simulink model "IEEE14_case"  (R2024b)
settings: Solver=FixedStepAuto  StartTime=0  StopTime=2  FixedStep=1e-7  RelTol=1e-3
values from neighbouring files (symbols this model uses):
  GFL_15_Bva = 0.009    [IEEE14_parameters.m]
  GFL_15_C_bus_pu = 7.179419    [IEEE14_parameters.m]
  GFL_15_f0 = 60    [IEEE14_parameters.m]
  GFL_15_I_id = 691.26967    [IEEE14_parameters.m]
  GFL_15_I_iq = 691.26967    [IEEE14_parameters.m]
  GFL_15_I_od = 45.2207    [IEEE14_parameters.m]
  GFL_15_I_oq = 45.2207    [IEEE14_parameters.m]
  GFL_15_I_pll = 0.78    [IEEE14_parameters.m]
  GFL_15_Kdi = 0.09    [IEEE14_parameters.m]
  GFL_15_Kdo = 0.9    [IEEE14_parameters.m]
  GFL_15_Kqi = 0.09    [IEEE14_parameters.m]
  GFL_15_Kqo = 0.9    [IEEE14_parameters.m]
  GFL_15_Lg_pu = 0.631447    [IEEE14_parameters.m]
  GFL_15_mode = 1    [IEEE14_parameters.m]
  GFL_15_P_id = 3.7166    [IEEE14_parameters.m]
  GFL_15_P_iq = 3.7166    [IEEE14_parameters.m]
  GFL_15_P_od = 0.4798    [IEEE14_parameters.m]
  GFL_15_P_oq = 0.4798    [IEEE14_parameters.m]
  GFL_15_P_pll = 290.42    [IEEE14_parameters.m]
  GFL_15_Qe_ref = 0.2    [IEEE14_parameters.m]
  GFL_15_Rg_pu = 0.024016    [IEEE14_parameters.m]
  GFL_15_Sbase = 1.000000e+4    (= 10000)    [IEEE14_parameters.m]
  GFL_15_Tdi = 0.01    [IEEE14_parameters.m]
  GFL_15_Tdo = 0.2    [IEEE14_parameters.m]
  GFL_15_Tqi = 0.01    [IEEE14_parameters.m]
  GFL_15_Tqo = 0.2    [IEEE14_parameters.m]
  GFL_15_Vbase = 380    [IEEE14_parameters.m]
  GFL_15_Vdc_ref = 1.011475    [IEEE14_parameters.m]
  GFL_15_Vdcbase = 700    [IEEE14_parameters.m]
  GFL_15_vq_ref = 0    [IEEE14_parameters.m]
  GFL_16_Bva = 0.002    [IEEE14_parameters.m]
  GFL_16_C_bus_pu = 7.179419    [IEEE14_parameters.m]
  GFL_16_f0 = 60    [IEEE14_parameters.m]
  GFL_16_I_id = 691.26967    [IEEE14_parameters.m]
  GFL_16_I_iq = 691.26967    [IEEE14_parameters.m]
  GFL_16_I_od = 45.2207    [IEEE14_parameters.m]
  GFL_16_I_oq = 45.2207    [IEEE14_parameters.m]
  GFL_16_I_pll = 0.78    [IEEE14_parameters.m]
  GFL_16_Kdi = 0.05    [IEEE14_parameters.m]
  GFL_16_Kdo = 0.5    [IEEE14_parameters.m]
  GFL_16_Kqi = 0.05    [IEEE14_parameters.m]
  GFL_16_Kqo = 0.5    [IEEE14_parameters.m]
  GFL_16_Lg_pu = 0.631447    [IEEE14_parameters.m]
  GFL_16_mode = 1    [IEEE14_parameters.m]
  GFL_16_P_id = 3.7166    [IEEE14_parameters.m]
  GFL_16_P_iq = 3.7166    [IEEE14_parameters.m]
  GFL_16_P_od = 0.4798    [IEEE14_parameters.m]
  GFL_16_P_oq = 0.4798    [IEEE14_parameters.m]
  GFL_16_P_pll = 290.42    [IEEE14_parameters.m]
  GFL_16_Qe_ref = 0.2    [IEEE14_parameters.m]
  GFL_16_Rg_pu = 0.024016    [IEEE14_parameters.m]
  GFL_16_Sbase = 1.000000e+4    (= 10000)    [IEEE14_parameters.m]
  GFL_16_Tdi = 0.01    [IEEE14_parameters.m]
  GFL_16_Tdo = 0.2    [IEEE14_parameters.m]
  GFL_16_Tqi = 0.01    [IEEE14_parameters.m]
  GFL_16_Tqo = 0.2    [IEEE14_parameters.m]
  GFL_16_Vbase = 380    [IEEE14_parameters.m]
  GFL_16_Vdc_ref = 1.01144    [IEEE14_parameters.m]
  GFL_16_Vdcbase = 700    [IEEE14_parameters.m]
  GFL_16_vq_ref = 0    [IEEE14_parameters.m]
  GFL_17_Bva = 0.002    [IEEE14_parameters.m]
  GFL_17_C_bus_pu = 7.179419    [IEEE14_parameters.m]
  GFL_17_f0 = 60    [IEEE14_parameters.m]
  GFL_17_I_id = 691.26967    [IEEE14_parameters.m]
  GFL_17_I_iq = 691.26967    [IEEE14_parameters.m]
  GFL_17_I_od = 45.2207    [IEEE14_parameters.m]
  GFL_17_I_oq = 45.2207    [IEEE14_parameters.m]
  GFL_17_I_pll = 0.78    [IEEE14_parameters.m]
  GFL_17_Kdi = 0.05    [IEEE14_parameters.m]
  GFL_17_Kdo = 0.5    [IEEE14_parameters.m]
  GFL_17_Kqi = 0.05    [IEEE14_parameters.m]
  GFL_17_Kqo = 0.5    [IEEE14_parameters.m]
  GFL_17_Lg_pu = 0.631447    [IEEE14_parameters.m]
  GFL_17_mode = 1    [IEEE14_parameters.m]
  GFL_17_P_id = 3.7166    [IEEE14_parameters.m]
  GFL_17_P_iq = 3.7166    [IEEE14_parameters.m]
  GFL_17_P_od = 0.4798    [IEEE14_parameters.m]
  GFL_17_P_oq = 0.4798    [IEEE14_parameters.m]
  GFL_17_P_pll = 290.42    [IEEE14_parameters.m]
  GFL_17_Qe_ref = 0.2    [IEEE14_parameters.m]
  GFL_17_Rg_pu = 0.024016    [IEEE14_parameters.m]
  GFL_17_Sbase = 1.000000e+4    (= 10000)    [IEEE14_parameters.m]
  GFL_17_Tdi = 0.01    [IEEE14_parameters.m]
  GFL_17_Tdo = 0.2    [IEEE14_parameters.m]
  GFL_17_Tqi = 0.01    [IEEE14_parameters.m]
  GFL_17_Tqo = 0.2    [IEEE14_parameters.m]
  GFL_17_Vbase = 380    [IEEE14_parameters.m]
  GFL_17_Vdc_ref = 1.011632    [IEEE14_parameters.m]
  GFL_17_Vdcbase = 700    [IEEE14_parameters.m]
  GFL_17_vq_ref = 0    [IEEE14_parameters.m]
  GFL_18_Bva = 0.002    [IEEE14_parameters.m]
  GFL_18_C_bus_pu = 7.179419    [IEEE14_parameters.m]
  GFL_18_f0 = 60    [IEEE14_parameters.m]
  GFL_18_I_id = 691.26967    [IEEE14_parameters.m]
  GFL_18_I_iq = 691.26967    [IEEE14_parameters.m]
  GFL_18_I_od = 45.2207    [IEEE14_parameters.m]
  GFL_18_I_oq = 45.2207    [IEEE14_parameters.m]
  GFL_18_I_pll = 0.78    [IEEE14_parameters.m]
  GFL_18_Kdi = 0.05    [IEEE14_parameters.m]
  GFL_18_Kdo = 0.5    [IEEE14_parameters.m]
  GFL_18_Kqi = 0.05    [IEEE14_parameters.m]
  GFL_18_Kqo = 0.5    [IEEE14_parameters.m]
  GFL_18_Lg_pu = 0.631447    [IEEE14_parameters.m]
  GFL_18_mode = 1    [IEEE14_parameters.m]
  GFL_18_P_id = 3.7166    [IEEE14_parameters.m]
  GFL_18_P_iq = 3.7166    [IEEE14_parameters.m]
  GFL_18_P_od = 0.4798    [IEEE14_parameters.m]
  GFL_18_P_oq = 0.4798    [IEEE14_parameters.m]
  GFL_18_P_pll = 290.42    [IEEE14_parameters.m]
  GFL_18_Qe_ref = 0.2    [IEEE14_parameters.m]
  GFL_18_Rg_pu = 0.024016    [IEEE14_parameters.m]
  GFL_18_Sbase = 1.000000e+4    (= 10000)    [IEEE14_parameters.m]
  GFL_18_Tdi = 0.01    [IEEE14_parameters.m]
  GFL_18_Tdo = 0.2    [IEEE14_parameters.m]
  GFL_18_Tqi = 0.01    [IEEE14_parameters.m]
  GFL_18_Tqo = 0.2    [IEEE14_parameters.m]
  GFL_18_Vbase = 380    [IEEE14_parameters.m]
  GFL_18_Vdc_ref = 1.011572    [IEEE14_parameters.m]
  GFL_18_Vdcbase = 700    [IEEE14_parameters.m]
  GFL_18_vq_ref = 0    [IEEE14_parameters.m]
  ... (+180 more)
(part 22 of 25)

== system IEEE14_case/SG_D_6/d_psi_fd_SG_D_6_block ==
  note: d_psi_fd_SG_D_6 in case14gfl
      | $-\frac{\psi _{\mathrm{fd},\mathrm{SG},D,6}-E_{\mathrm{fd},\mathrm{SG},D,6}+\left(x_{d}-x_{\mathrm{dd}}\right)\,\left(\frac{\frac{\psi _{\mathrm{1d},\mathrm{SG},D,6}\,\left(x_{\mathrm{dd}}-x_{\mathrm{ddd}}\right)}{x_{\mathrm{dd}}-x_{l}}-\psi _{d,\mathrm{SG},D,6}+\frac{\psi _{\mathrm{fd},\mathrm{SG},D,6}\,\left(x_{\mathrm{ddd}}-x_{l}\right)}{x_{\mathrm{dd}}-x_{l}}}{x_{\mathrm{ddd}}}-\frac{\left(x_{\mathrm{dd}}-x_{\mathrm{ddd}}\right)\,\left(\psi _{\mathrm{1d},\mathrm{SG},D,6}-\psi _{\mathrm{fd},\mathrm{SG},D,6}+\frac{\left(x_{\mathrm{dd}}-x_{l}\right)\,\left(\frac{\psi _{\mathrm{1d},\mathrm{SG},D,6}\,\left(x_{\mathrm{dd}}-x_{\mathrm{ddd}}\right)}{x_{\mathrm{dd}}-x_{l}}-\psi _{d,\mathrm{SG},D,6}+\frac{\psi _{\mathrm{fd},\mathrm{SG},D,6}\,\left(x_{\mathrm{ddd}}-x_{l}\right)}{x_{\mathrm{dd}}-x_{l}}\right)}{x_{\mathrm{ddd}}}\right)}{{\left(x_{\mathrm{dd}}-x_{l}\right)}^2}\right)}{T_{\mathrm{dd}}}$
      | Automatically generated on 2025-10-09 21:32:58 .
  State_E_fd_SG_D_6_8c2c7 : Inport
  State_psi_fd_SG_D_6_cff00 : Inport  Port=2
  State_psi_1d_SG_D_6_bc672 : Inport  Port=3
  State_psi_fd_SG_D_6_4e3f4 : Inport  Port=4
  State_psi_1d_SG_D_6_ebde4 : Inport  Port=5
  State_psi_d_SG_D_6_92222 : Inport  Port=6
  State_psi_fd_SG_D_6_38b04 : Inport  Port=7
  State_psi_1d_SG_D_6_32df7 : Inport  Port=8
  State_psi_d_SG_D_6_beaed : Inport  Port=9
  State_psi_fd_SG_D_6_10d72 : Inport  Port=10
  Add_ba2f2 : Sum
  Add_cdb5d : Sum
  Constant_-1_792aa : Constant  Value=-1
  Constant_-1_a3724 : Constant  Value=-1
  Constant_-1_f4132 : Constant  Value=-1
  Constant_2.0_0b013 : Constant  Value=2.0
  Constant_T_dd_62463 : Constant  Value=T_dd
  Constant_x_d_b318c : Constant  Value=x_d
  Constant_x_dd_0a587 : Constant  Value=x_dd
  Constant_x_dd_2d805 : Constant  Value=x_dd
  Constant_x_dd_68d39 : Constant  Value=x_dd
  Constant_x_dd_81c4f : Constant  Value=x_dd
  Constant_x_dd_82b55 : Constant  Value=x_dd
  Constant_x_dd_8a32d : Constant  Value=x_dd
  Constant_x_dd_b822f : Constant  Value=x_dd
  Constant_x_dd_ddb07 : Constant  Value=x_dd
  Constant_x_dd_f11c0 : Constant  Value=x_dd
  Constant_x_dd_fd22e : Constant  Value=x_dd
  Constant_x_ddd_04df1 : Constant  Value=x_ddd
  Constant_x_ddd_0bc83 : Constant  Value=x_ddd
  Constant_x_ddd_0c2e6 : Constant  Value=x_ddd
  Constant_x_ddd_68b46 : Constant  Value=x_ddd
  Constant_x_ddd_9c9d7 : Constant  Value=x_ddd
  Constant_x_ddd_b1a79 : Constant  Value=x_ddd
  Constant_x_ddd_f3fb2 : Constant  Value=x_ddd
  Constant_x_l_2e508 : Constant  Value=x_l
  Constant_x_l_329a5 : Constant  Value=x_l
  Constant_x_l_400bf : Constant  Value=x_l
  Constant_x_l_84374 : Constant  Value=x_l
  Constant_x_l_978cf : Constant  Value=x_l
  Constant_x_l_b454b : Constant  Value=x_l
  Constant_x_l_d1dca : Constant  Value=x_l
  Constant_x_l_deb57 : Constant  Value=x_l
  Divide_172f0 : Product  Inputs=*/
  Divide_302a3 : Product  Inputs=*/
  Divide_32902 : Product  Inputs=*/
  Divide_a0797 : Product  Inputs=*/
  Divide_ab6db : Product  Inputs=*/
  Divide_b1b26 : Product  Inputs=*/
  Divide_d407a : Product  Inputs=*/
  Divide_da2d9 : Product  Inputs=*/
  Power_b35c3 : Math  Operator=pow
  Product_04d90 : Product
  Product_25107 : Product
  Product_3678f : Product
  Product_38c26 : Product
  Product_4f01a : Product
  Product_8b753 : Product
  Product_9bbf1 : Product
  Product_adb41 : Product
  Product_f7c34 : Product
  Product_fcd24 : Product
  Subtract_088af : Sum  Inputs=+-
  Subtract_0a0c0 : Sum  Inputs=+-
  Subtract_0b103 : Sum  Inputs=+-
  Subtract_121da : Sum  Inputs=+-
  Subtract_441e5 : Sum  Inputs=+-
  Subtract_539cc : Sum  Inputs=+-
  Subtract_59274 : Sum  Inputs=+-
  Subtract_66fab : Sum  Inputs=+-
  Subtract_6b641 : Sum  Inputs=+-
  Subtract_8929d : Sum  Inputs=+-
  Subtract_8cd83 : Sum  Inputs=+-
  Subtract_8e7ae : Sum  Inputs=+-
  Subtract_923ad : Sum  Inputs=+-
  Subtract_9258f : Sum  Inputs=+-
  Subtract_960a4 : Sum  Inputs=+-
  Subtract_a221f : Sum  Inputs=+-
  Subtract_bcf8f : Sum  Inputs=+-
  Subtract_daa8f : Sum  Inputs=+-
  Subtract_e7b9f : Sum  Inputs=+-
  Blockout_d_psi_fd_SG_D_6_50674 : Outport
  wires:
  Constant_-1_a3724/1 -> Product_8b753/1
  Constant_x_l_329a5/1 -> Subtract_121da/2
  Constant_x_dd_0a587/1 -> Subtract_0a0c0/1
  State_psi_1d_SG_D_6_ebde4/1 -> Product_8b753/2
  Constant_x_dd_8a32d/1 -> Subtract_088af/1
  Subtract_59274/1 -> Product_25107/2
  Constant_x_ddd_b1a79/1 -> Subtract_0a0c0/2
  Constant_-1_792aa/1 -> Product_9bbf1/1
  Product_8b753/1 -> Product_f7c34/1
  Constant_x_dd_b822f/1 -> Subtract_0b103/1
  Constant_x_l_978cf/1 -> Subtract_66fab/2
  Subtract_0a0c0/1 -> Product_f7c34/2
  Constant_x_l_2e508/1 -> Subtract_088af/2
  Subtract_960a4/1 -> Product_adb41/2
  Constant_x_ddd_0bc83/1 -> Subtract_960a4/1
  Constant_x_l_deb57/1 -> Subtract_960a4/2
  Product_f7c34/1 -> Divide_d407a/1
  Constant_x_dd_2d805/1 -> Subtract_9258f/1
  Subtract_088af/1 -> Divide_d407a/2
  State_psi_fd_SG_D_6_38b04/1 -> Product_adb41/1
  Subtract_8e7ae/1 -> Product_3678f/1
  Constant_x_dd_f11c0/1 -> Subtract_121da/1
  Constant_T_dd_62463/1 -> Divide_32902/2
  State_psi_1d_SG_D_6_bc672/1 -> Subtract_e7b9f/1
  Divide_d407a/1 -> Add_cdb5d/1
  Product_38c26/1 -> Divide_302a3/1
  Divide_172f0/1 -> Subtract_8cd83/2
  State_psi_d_SG_D_6_92222/1 -> Add_cdb5d/2
  Product_adb41/1 -> Divide_172f0/1
  Subtract_121da/1 -> Divide_172f0/2
  Constant_x_dd_68d39/1 -> Subtract_8e7ae/1
  Constant_x_l_84374/1 -> Subtract_8e7ae/2
  Add_cdb5d/1 -> Subtract_8cd83/1
  Subtract_e7b9f/1 -> Subtract_539cc/1
  State_psi_1d_SG_D_6_32df7/1 -> Product_9bbf1/2
  Constant_x_ddd_0c2e6/1 -> Subtract_0b103/2
  Subtract_8cd83/1 -> Product_3678f/2
  Product_9bbf1/1 -> Product_4f01a/1
  Subtract_0b103/1 -> Product_4f01a/2
  Subtract_441e5/1 -> Product_38c26/2
  Constant_x_l_b454b/1 -> Subtract_9258f/2
  Constant_x_ddd_68b46/1 -> Subtract_441e5/1
  Constant_x_l_400bf/1 -> Subtract_441e5/2
  State_psi_d_SG_D_6_beaed/1 -> Add_ba2f2/2
  Constant_x_dd_ddb07/1 -> Subtract_59274/1
  Constant_x_ddd_f3fb2/1 -> Subtract_59274/2
  Constant_x_dd_fd22e/1 -> Subtract_8929d/1
  State_psi_fd_SG_D_6_4e3f4/1 -> Subtract_e7b9f/2
  Product_3678f/1 -> Divide_ab6db/1
  Constant_x_ddd_9c9d7/1 -> Divide_ab6db/2
  Product_4f01a/1 -> Divide_da2d9/1
  Subtract_9258f/1 -> Divide_da2d9/2
  State_psi_fd_SG_D_6_10d72/1 -> Product_38c26/1
  Constant_x_dd_82b55/1 -> Subtract_66fab/1
  Constant_-1_f4132/1 -> Product_25107/1
  Divide_ab6db/1 -> Subtract_539cc/2
  Product_25107/1 -> Product_fcd24/1
  Divide_da2d9/1 -> Add_ba2f2/1
  Constant_x_l_d1dca/1 -> Subtract_8929d/2
  Subtract_66fab/1 -> Divide_302a3/2
  Subtract_539cc/1 -> Product_fcd24/2
  Subtract_8929d/1 -> Power_b35c3/1
  Constant_2.0_0b013/1 -> Power_b35c3/2
  Add_ba2f2/1 -> Subtract_bcf8f/1
  Divide_302a3/1 -> Subtract_bcf8f/2
  Product_fcd24/1 -> Divide_b1b26/1
  Power_b35c3/1 -> Divide_b1b26/2
  Subtract_bcf8f/1 -> Divide_a0797/1
  Constant_x_ddd_04df1/1 -> Divide_a0797/2
  Constant_x_d_b318c/1 -> Subtract_daa8f/1
  Constant_x_dd_81c4f/1 -> Subtract_daa8f/2
  Divide_b1b26/1 -> Subtract_6b641/1
  Divide_a0797/1 -> Subtract_6b641/2
  State_E_fd_SG_D_6_8c2c7/1 -> Subtract_923ad/1
  State_psi_fd_SG_D_6_cff00/1 -> Subtract_923ad/2
  Subtract_daa8f/1 -> Product_04d90/1
  Subtract_6b641/1 -> Product_04d90/2
  Subtract_923ad/1 -> Subtract_a221f/1
  Product_04d90/1 -> Subtract_a221f/2
  Subtract_a221f/1 -> Divide_32902/1
  Divide_32902/1 -> Blockout_d_psi_fd_SG_D_6_50674/1

== system IEEE14_case/SG_D_6/d_psi_gq_SG_D_6_block ==
  note: d_psi_gq_SG_D_6 in case14gfl
      | $-\frac{\psi _{\mathrm{gq},\mathrm{SG},D,6}+\left(x_{q}-x_{\mathrm{qd}}\right)\,\left(\frac{\psi _{q,\mathrm{SG},D,6}+\frac{\psi _{\mathrm{gq},\mathrm{SG},D,6}\,\left(x_{l}-x_{\mathrm{qdd}}\right)}{x_{l}-x_{\mathrm{qd}}}+\frac{\psi _{\mathrm{kq},\mathrm{SG},D,6}\,\left(x_{\mathrm{qd}}-x_{\mathrm{qdd}}\right)}{x_{l}-x_{\mathrm{qd}}}}{x_{\mathrm{qdd}}}+\frac{\left(x_{\mathrm{qd}}-x_{\mathrm{qdd}}\right)\,\left(\psi _{\mathrm{gq},\mathrm{SG},D,6}+\psi _{\mathrm{kq},\mathrm{SG},D,6}+\frac{\left(x_{l}-x_{\mathrm{qd}}\right)\,\left(\psi _{q,\mathrm{SG},D,6}+\frac{\psi _{\mathrm{gq},\mathrm{SG},D,6}\,\left(x_{l}-x_{\mathrm{qdd}}\right)}{x_{l}-x_{\mathrm{qd}}}+\frac{\psi _{\mathrm{kq},\mathrm{SG},D,6}\,\left(x_{\mathrm{qd}}-x_{\mathrm{qdd}}\right)}{x_{l}-x_{\mathrm{qd}}}\right)}{x_{\mathrm{qdd}}}\right)}{{\left(x_{l}-x_{\mathrm{qd}}\right)}^2}\right)}{T_{\mathrm{qd}}}$
      | Automatically generated on 2025-10-09 21:33:06 .
  State_psi_gq_SG_D_6_9681f : Inport
  State_psi_gq_SG_D_6_f7256 : Inport  Port=2
  State_psi_kq_SG_D_6_591fc : Inport  Port=3
  State_psi_gq_SG_D_6_8e9c1 : Inport  Port=4
  State_psi_kq_SG_D_6_f7f8f : Inport  Port=5
  State_psi_q_SG_D_6_acf1b : Inport  Port=6
  State_psi_gq_SG_D_6_45442 : Inport  Port=7
  State_psi_kq_SG_D_6_32c36 : Inport  Port=8
  State_psi_q_SG_D_6_63591 : Inport  Port=9
  Add_0385f : Sum
  Add_2fca8 : Sum
  Add_45bb5 : Sum
  Add_4fe74 : Sum
  Add_6652c : Sum
  Add_72abd : Sum
  Add_ab6e5 : Sum
  Add_b3e8e : Sum
  Add_d55a4 : Sum
  Add_ddfd3 : Sum
  Add_e44b6 : Sum
  Add_e85b8 : Sum
  Constant_-1_02a2b : Constant  Value=-1
  Constant_-1_0cf12 : Constant  Value=-1
  Constant_-1_338a9 : Constant  Value=-1
  Constant_-1_4b5b4 : Constant  Value=-1
  Constant_-1_77f81 : Constant  Value=-1
  Constant_-1_7e2c9 : Constant  Value=-1
  Constant_-1_a0540 : Constant  Value=-1
  Constant_-1_a4fbb : Constant  Value=-1
  Constant_-1_ab8f6 : Constant  Value=-1
  Constant_-1_f6b01 : Constant  Value=-1
  Constant_2.0_57b4a : Constant  Value=2.0
  Constant_T_qd_232d6 : Constant  Value=T_qd
  Constant_x_l_3f2c2 : Constant  Value=x_l
  Constant_x_l_6be57 : Constant  Value=x_l
  Constant_x_l_70d85 : Constant  Value=x_l
  Constant_x_l_b3499 : Constant  Value=x_l
  Constant_x_l_c674e : Constant  Value=x_l
  Constant_x_l_d8074 : Constant  Value=x_l
  Constant_x_l_f4412 : Constant  Value=x_l
  Constant_x_l_feb5e : Constant  Value=x_l
  Constant_x_q_1f822 : Constant  Value=x_q
  Constant_x_qd_0f880 : Constant  Value=x_qd
  Constant_x_qd_265a1 : Constant  Value=x_qd
  Constant_x_qd_28a79 : Constant  Value=x_qd
  Constant_x_qd_2fba1 : Constant  Value=x_qd
  Constant_x_qd_3d557 : Constant  Value=x_qd
  Constant_x_qd_5e447 : Constant  Value=x_qd
  Constant_x_qd_a1d86 : Constant  Value=x_qd
  Constant_x_qd_a2469 : Constant  Value=x_qd
  Constant_x_qd_c046f : Constant  Value=x_qd
  Constant_x_qd_e5b71 : Constant  Value=x_qd
  Constant_x_qdd_04dbe : Constant  Value=x_qdd
  Constant_x_qdd_0de89 : Constant  Value=x_qdd
  Constant_x_qdd_13ba8 : Constant  Value=x_qdd
  Constant_x_qdd_30e2b : Constant  Value=x_qdd
  Constant_x_qdd_7bfd7 : Constant  Value=x_qdd
  Constant_x_qdd_8d34f : Constant  Value=x_qdd
  Constant_x_qdd_bdf93 : Constant  Value=x_qdd
  Divide_048c6 : Product  Inputs=*/
  Divide_20769 : Product  Inputs=*/
  Divide_4620f : Product  Inputs=*/
  Divide_5fb59 : Product  Inputs=*/
  Divide_62d2e : Product  Inputs=*/
  Divide_ad365 : Product  Inputs=*/
  Divide_b0aab : Product  Inputs=*/
  Divide_b5ca2 : Product  Inputs=*/
  Power_de08a : Math  Operator=pow
  Product_0c41a : Product
  Product_1bf10 : Product
  Product_21034 : Product
  Product_21968 : Product
  Product_35c5d : Product
  Product_4f086 : Product
  Product_5c9ea : Product
  Product_5cf60 : Product
  Product_85043 : Product
  Product_8afed : Product
  Product_8ed51 : Product
  Product_a9aa3 : Product
  Product_b6c44 : Product
  Product_d191a : Product
  Product_d321a : Product
  Product_daf4d : Product
  Product_e22b9 : Product
  Subtract_52724 : Sum  Inputs=+-
  Subtract_5a596 : Sum  Inputs=+-
  Subtract_8624a : Sum  Inputs=+-
  Subtract_8bdeb : Sum  Inputs=+-
  Subtract_8cbf2 : Sum  Inputs=+-
  Subtract_a120b : Sum  Inputs=+-
  Subtract_ac106 : Sum  Inputs=+-
  Subtract_cce7d : Sum  Inputs=+-
  Blockout_d_psi_gq_SG_D_6_58558 : Outport
  wires:
  Constant_-1_a4fbb/1 -> Product_8ed51/1
  Constant_x_l_70d85/1 -> Product_d321a/2
  Constant_x_l_feb5e/1 -> Product_0c41a/2
  Constant_x_qd_0f880/1 -> Subtract_8bdeb/1
  Constant_-1_f6b01/1 -> Product_b6c44/1
  Constant_x_qdd_7bfd7/1 -> Add_4fe74/2
  Constant_x_qdd_8d34f/1 -> Subtract_8cbf2/2
  Constant_x_qd_3d557/1 -> Add_ab6e5/2
  Constant_-1_7e2c9/1 -> Product_21968/1
  Constant_x_qdd_13ba8/1 -> Subtract_8bdeb/2
  Constant_x_l_f4412/1 -> Product_21968/2
  Constant_x_l_6be57/1 -> Product_a9aa3/2
  Product_21968/1 -> Add_4fe74/1
  Product_d321a/1 -> Add_e85b8/1
  Constant_-1_ab8f6/1 -> Product_0c41a/1
  Constant_x_l_3f2c2/1 -> Product_b6c44/2
  Constant_x_qd_a2469/1 -> Add_e44b6/2
  State_psi_gq_SG_D_6_8e9c1/1 -> Product_4f086/1
  Add_4fe74/1 -> Product_4f086/2
  Product_0c41a/1 -> Add_6652c/1
  Add_45bb5/1 -> Subtract_52724/1
  Constant_x_qdd_30e2b/1 -> Add_e85b8/2
  Constant_x_qd_5e447/1 -> Add_6652c/2
  Product_daf4d/1 -> Add_d55a4/1
  State_psi_kq_SG_D_6_f7f8f/1 -> Product_1bf10/1
  Subtract_8bdeb/1 -> Product_1bf10/2
  State_psi_kq_SG_D_6_32c36/1 -> Product_85043/1
  Product_b6c44/1 -> Add_ab6e5/1
  Product_4f086/1 -> Divide_b0aab/1
  Add_6652c/1 -> Divide_b0aab/2
  Product_1bf10/1 -> Divide_ad365/1
  State_psi_gq_SG_D_6_f7256/1 -> Add_45bb5/1
  Add_ab6e5/1 -> Divide_ad365/2
  Constant_x_l_b3499/1 -> Product_5cf60/2
  Constant_-1_0cf12/1 -> Product_a9aa3/1
  Divide_b0aab/1 -> Subtract_a120b/1
  Divide_ad365/1 -> Subtract_a120b/2
  State_psi_kq_SG_D_6_591fc/1 -> Add_45bb5/2
  Constant_-1_a0540/1 -> Product_d321a/1
  Product_a9aa3/1 -> Add_b3e8e/1
  Constant_x_qd_265a1/1 -> Add_b3e8e/2
  Subtract_a120b/1 -> Add_ddfd3/1
  State_psi_q_SG_D_6_acf1b/1 -> Add_ddfd3/2
  Constant_x_qd_e5b71/1 -> Subtract_ac106/1
  Constant_-1_02a2b/1 -> Product_daf4d/1
  Add_d55a4/1 -> Divide_5fb59/2
  Constant_x_l_d8074/1 -> Product_daf4d/2
  Constant_x_qd_a1d86/1 -> Subtract_8cbf2/1
  Constant_-1_77f81/1 -> Product_d191a/1
  Constant_x_l_c674e/1 -> Product_d191a/2
  Add_b3e8e/1 -> Product_5c9ea/1
  Constant_-1_338a9/1 -> Product_5cf60/1
  Subtract_cce7d/1 -> Product_21034/2
  Constant_x_qdd_0de89/1 -> Subtract_ac106/2
  Add_ddfd3/1 -> Product_5c9ea/2
  State_psi_gq_SG_D_6_45442/1 -> Product_8afed/1
  Add_e85b8/1 -> Product_8afed/2
  Constant_x_qd_2fba1/1 -> Add_d55a4/2
  Subtract_8cbf2/1 -> Product_85043/2
  Product_d191a/1 -> Add_e44b6/1
  Product_5c9ea/1 -> Divide_048c6/1
  Constant_x_qdd_04dbe/1 -> Divide_048c6/2
  Product_8afed/1 -> Divide_5fb59/1
  Product_85043/1 -> Divide_62d2e/1
  Add_e44b6/1 -> Divide_62d2e/2
  Constant_x_qd_c046f/1 -> Add_0385f/2
  Subtract_ac106/1 -> Product_8ed51/2
  Divide_048c6/1 -> Subtract_52724/2
  Product_5cf60/1 -> Add_0385f/1
  Divide_5fb59/1 -> Subtract_8624a/1
  Divide_62d2e/1 -> Subtract_8624a/2
  Product_8ed51/1 -> Product_35c5d/1
  Subtract_52724/1 -> Product_35c5d/2
  Add_0385f/1 -> Power_de08a/1
  Constant_2.0_57b4a/1 -> Power_de08a/2
  Subtract_8624a/1 -> Add_72abd/1
  State_psi_q_SG_D_6_63591/1 -> Add_72abd/2
  Product_35c5d/1 -> Divide_4620f/1
  Power_de08a/1 -> Divide_4620f/2
  Add_72abd/1 -> Divide_b5ca2/1
  Constant_x_qdd_bdf93/1 -> Divide_b5ca2/2
  Constant_x_q_1f822/1 -> Subtract_5a596/1
  Constant_x_qd_28a79/1 -> Subtract_5a596/2
  Divide_4620f/1 -> Subtract_cce7d/1
  Divide_b5ca2/1 -> Subtract_cce7d/2
  Constant_-1_4b5b4/1 -> Product_e22b9/1
  State_psi_gq_SG_D_6_9681f/1 -> Product_e22b9/2
  Subtract_5a596/1 -> Product_21034/1
  Product_e22b9/1 -> Add_2fca8/1
  Product_21034/1 -> Add_2fca8/2
  Add_2fca8/1 -> Divide_20769/1
  Divide_20769/1 -> Blockout_d_psi_gq_SG_D_6_58558/1
  Constant_T_qd_232d6/1 -> Divide_20769/2

== system IEEE14_case/SG_D_6/d_psi_kq_SG_D_6_block ==
  note: d_psi_kq_SG_D_6 in case14gfl
      | $-\frac{\psi _{\mathrm{gq},\mathrm{SG},D,6}+\psi _{\mathrm{kq},\mathrm{SG},D,6}+\frac{\left(x_{l}-x_{\mathrm{qd}}\right)\,\left(\psi _{q,\mathrm{SG},D,6}+\frac{\psi _{\mathrm{gq},\mathrm{SG},D,6}\,\left(x_{l}-x_{\mathrm{qdd}}\right)}{x_{l}-x_{\mathrm{qd}}}+\frac{\psi _{\mathrm{kq},\mathrm{SG},D,6}\,\left(x_{\mathrm{qd}}-x_{\mathrm{qdd}}\right)}{x_{l}-x_{\mathrm{qd}}}\right)}{x_{\mathrm{qdd}}}}{T_{\mathrm{qdd}}}$
      | Automatically generated on 2025-10-09 21:33:09 .
  State_psi_gq_SG_D_6_1d13a : Inport
  State_psi_kq_SG_D_6_a092f : Inport  Port=2
  State_psi_gq_SG_D_6_38b04 : Inport  Port=3
  State_psi_kq_SG_D_6_0165b : Inport  Port=4
  State_psi_q_SG_D_6_e39b7 : Inport  Port=5
  Add_3dba8 : Sum
  Add_90f35 : Sum
  Add_9e227 : Sum
  Add_c159c : Sum
  Add_e2562 : Sum
  Add_e5c09 : Sum
  Constant_-1_0a0f1 : Constant  Value=-1
  Constant_-1_84daa : Constant  Value=-1
  Constant_-1_b779e : Constant  Value=-1
  Constant_-1_bf8d5 : Constant  Value=-1
  Constant_-1_da0f3 : Constant  Value=-1
  Constant_T_qdd_8dbb6 : Constant  Value=T_qdd
  Constant_x_l_30299 : Constant  Value=x_l
  Constant_x_l_33695 : Constant  Value=x_l
  Constant_x_l_c7a15 : Constant  Value=x_l
  Constant_x_l_f8f06 : Constant  Value=x_l
  Constant_x_qd_38861 : Constant  Value=x_qd
  Constant_x_qd_63e92 : Constant  Value=x_qd
  Constant_x_qd_6749d : Constant  Value=x_qd
  Constant_x_qd_c986d : Constant  Value=x_qd
  Constant_x_qdd_77268 : Constant  Value=x_qdd
  Constant_x_qdd_db300 : Constant  Value=x_qdd
  Constant_x_qdd_e5bf2 : Constant  Value=x_qdd
  Divide_1415c : Product  Inputs=*/
  Divide_47c01 : Product  Inputs=*/
  Divide_bfe60 : Product  Inputs=*/
  Divide_d58ce : Product  Inputs=*/
  Product_2db5e : Product
  Product_831e3 : Product
  Product_8d51a : Product
  Product_92199 : Product
  Product_a451d : Product
  Product_a8b7d : Product
  Product_bdb4f : Product
  Product_f40fe : Product
  Subtract_0ef18 : Sum  Inputs=+-
  Subtract_427cd : Sum  Inputs=+-
  Subtract_bed08 : Sum  Inputs=+-
  Blockout_d_psi_kq_SG_D_6_f15a3 : Outport
  wires:
  Constant_x_qd_c986d/1 -> Add_c159c/2
  Constant_-1_bf8d5/1 -> Product_f40fe/1
  Constant_-1_0a0f1/1 -> Product_92199/1
  Constant_-1_da0f3/1 -> Product_bdb4f/1
  Constant_x_qd_63e92/1 -> Subtract_0ef18/1
  Product_f40fe/1 -> Add_90f35/1
  Constant_x_l_f8f06/1 -> Product_92199/2
  Constant_T_qdd_8dbb6/1 -> Divide_1415c/2
  Constant_x_qdd_77268/1 -> Add_90f35/2
  Constant_x_l_c7a15/1 -> Product_f40fe/2
  Constant_x_qdd_db300/1 -> Subtract_0ef18/2
  Constant_-1_b779e/1 -> Product_a451d/1
  Constant_x_l_30299/1 -> Product_a451d/2
  State_psi_gq_SG_D_6_38b04/1 -> Product_a8b7d/1
  State_psi_kq_SG_D_6_a092f/1 -> Subtract_427cd/2
  Add_90f35/1 -> Product_a8b7d/2
  Divide_d58ce/1 -> Subtract_bed08/1
  Product_92199/1 -> Add_c159c/1
  Subtract_427cd/1 -> Add_e5c09/1
  State_psi_kq_SG_D_6_0165b/1 -> Product_831e3/1
  Subtract_0ef18/1 -> Product_831e3/2
  Product_2db5e/1 -> Divide_bfe60/1
  Product_a451d/1 -> Add_9e227/1
  Constant_x_qd_6749d/1 -> Add_9e227/2
  Product_a8b7d/1 -> Divide_d58ce/1
  Add_c159c/1 -> Divide_d58ce/2
  Product_831e3/1 -> Divide_47c01/1
  Add_9e227/1 -> Divide_47c01/2
  Constant_x_l_33695/1 -> Product_bdb4f/2
  Subtract_bed08/1 -> Add_3dba8/1
  Divide_47c01/1 -> Subtract_bed08/2
  Product_bdb4f/1 -> Add_e2562/1
  Constant_x_qd_38861/1 -> Add_e2562/2
  State_psi_q_SG_D_6_e39b7/1 -> Add_3dba8/2
  Constant_-1_84daa/1 -> Product_8d51a/1
  State_psi_gq_SG_D_6_1d13a/1 -> Product_8d51a/2
  Add_e2562/1 -> Product_2db5e/1
  Add_3dba8/1 -> Product_2db5e/2
  Product_8d51a/1 -> Subtract_427cd/1
  Divide_1415c/1 -> Blockout_d_psi_kq_SG_D_6_f15a3/1
  Constant_x_qdd_e5bf2/1 -> Divide_bfe60/2
  Divide_bfe60/1 -> Add_e5c09/2
  Add_e5c09/1 -> Divide_1415c/1

== system IEEE14_case/SG_D_6/d_psi_q_SG_D_6_block ==
  note: d_psi_q_SG_D_6 in case14gfl
      | $2\,\pi \,f_{0}\,\left(v_{d,\mathrm{SG},D,6}\,\cos\left(\theta _{\mathrm{SG},D,6}\right)+v_{q,\mathrm{SG},D,6}\,\sin\left(\theta _{\mathrm{SG},D,6}\right)-\frac{R_{a}\,\left(\psi _{q,\mathrm{SG},D,6}+\frac{\psi _{\mathrm{gq},\mathrm{SG},D,6}\,\left(x_{l}-x_{\mathrm{qdd}}\right)}{x_{l}-x_{\mathrm{qd}}}+\frac{\psi _{\mathrm{kq},\mathrm{SG},D,6}\,\left(x_{\mathrm{qd}}-x_{\mathrm{qdd}}\right)}{x_{l}-x_{\mathrm{qd}}}\right)}{x_{\mathrm{qdd}}}-\frac{\psi _{d,\mathrm{SG},D,6}\,w_{\mathrm{SG},D,6}}{2\,f_{0}\,\pi }\right)$
      | Automatically generated on 2025-10-09 21:32:54 .
  State_psi_gq_SG_D_6_ae354 : Inport
  State_psi_kq_SG_D_6_fbd08 : Inport  Port=2
  State_psi_q_SG_D_6_163e7 : Inport  Port=3
  Input_v_d_SG_D_6_c50dc : Inport  Port=4
  State_theta_SG_D_6_a7791 : Inport  Port=5
  Input_v_q_SG_D_6_f6a8c : Inport  Port=6
  State_theta_SG_D_6_9e13e : Inport  Port=7
  State_psi_d_SG_D_6_700ce : Inport  Port=8
  State_w_SG_D_6_19237 : Inport  Port=9
  Add_014fe : Sum
  Add_143fb : Sum
  Add_f55ab : Sum
  Add_f7332 : Sum
  Add_fe05f : Sum
  Constant_-1_2a46f : Constant  Value=-1
  Constant_-1_5aef8 : Constant  Value=-1
  Constant_-1_b7296 : Constant  Value=-1
  Constant_-2.0_6bd1f : Constant  Value=-2.0
  Constant_2.0_827e2 : Constant  Value=2.0
  Constant_R_a_3af7e : Constant  Value=R_a
  Constant_f0_c27e4 : Constant  Value=f0
  Constant_f0_dce12 : Constant  Value=f0
  Constant_pi_d58e0 : Constant  Value=pi
  Constant_pi_dab8a : Constant  Value=pi
  Constant_x_l_23d60 : Constant  Value=x_l
  Constant_x_l_6d18d : Constant  Value=x_l
  Constant_x_l_9160c : Constant  Value=x_l
  Constant_x_qd_7b1ad : Constant  Value=x_qd
  Constant_x_qd_ebf67 : Constant  Value=x_qd
  Constant_x_qd_f3e4e : Constant  Value=x_qd
  Constant_x_qdd_1fc71 : Constant  Value=x_qdd
  Constant_x_qdd_44ed9 : Constant  Value=x_qdd
  Constant_x_qdd_a155d : Constant  Value=x_qdd
  Divide_08384 : Product  Inputs=*/
  Divide_1b459 : Product  Inputs=*/
  Divide_97fe9 : Product  Inputs=*/
  Divide_fd7a5 : Product  Inputs=*/
  MathFunc_cos_41055 : Trigonometry  Operator=cos
  MathFunc_sin_66cc9 : Trigonometry
  Product_055b8 : Product
  Product_08fcd : Product
  Product_0d753 : Product
  Product_23c04 : Product
  Product_23c87 : Product
  Product_328fc : Product
  Product_37e9e : Product
  Product_43aa7 : Product
  Product_6be21 : Product
  Product_6d514 : Product
  Product_6e059 : Product
  Product_75a8f : Product
  Product_9e638 : Product
  Product_b1887 : Product
  Subtract_2d9ef : Sum  Inputs=+-
  Subtract_75a6e : Sum  Inputs=+-
  Subtract_988de : Sum  Inputs=+-
  Subtract_f81ea : Sum  Inputs=+-
  Blockout_d_psi_q_SG_D_6_609ad : Outport
  wires:
  Constant_x_qd_f3e4e/1 -> Subtract_f81ea/1
  Product_37e9e/1 -> Divide_1b459/1
  Constant_-1_5aef8/1 -> Product_6e059/1
  Constant_-2.0_6bd1f/1 -> Product_6be21/1
  Input_v_d_SG_D_6_c50dc/1 -> Product_9e638/1
  Constant_x_qdd_a155d/1 -> Subtract_f81ea/2
  Constant_x_l_23d60/1 -> Product_6e059/2
  Constant_f0_dce12/1 -> Product_43aa7/2
  Constant_pi_d58e0/1 -> Product_328fc/2
  Product_6d514/1 -> Divide_fd7a5/1
  Product_6e059/1 -> Add_f7332/1
  Constant_x_l_9160c/1 -> Product_75a8f/2
  Product_23c87/1 -> Divide_1b459/2
  State_w_SG_D_6_19237/1 -> Product_37e9e/2
  Add_f55ab/1 -> Divide_97fe9/2
  Constant_x_qdd_1fc71/1 -> Add_f7332/2
  Constant_2.0_827e2/1 -> Product_328fc/1
  Add_143fb/1 -> Product_6d514/2
  Constant_-1_b7296/1 -> Product_75a8f/1
  Constant_-1_2a46f/1 -> Product_055b8/1
  Constant_x_l_6d18d/1 -> Product_055b8/2
  State_theta_SG_D_6_9e13e/1 -> MathFunc_sin_66cc9/1
  State_psi_gq_SG_D_6_ae354/1 -> Product_0d753/1
  Add_f7332/1 -> Product_0d753/2
  Product_328fc/1 -> Product_23c87/1
  Product_75a8f/1 -> Add_f55ab/1
  Subtract_75a6e/1 -> Add_fe05f/1
  Constant_f0_c27e4/1 -> Product_23c87/2
  MathFunc_sin_66cc9/1 -> Product_b1887/2
  Product_0d753/1 -> Divide_97fe9/1
  Constant_x_qd_7b1ad/1 -> Add_f55ab/2
  State_psi_kq_SG_D_6_fbd08/1 -> Product_08fcd/1
  Subtract_f81ea/1 -> Product_08fcd/2
  Product_055b8/1 -> Add_014fe/1
  Constant_x_qd_ebf67/1 -> Add_014fe/2
  Product_08fcd/1 -> Divide_08384/1
  Constant_x_qdd_44ed9/1 -> Divide_fd7a5/2
  Add_014fe/1 -> Divide_08384/2
  Divide_97fe9/1 -> Subtract_2d9ef/1
  Subtract_2d9ef/1 -> Add_143fb/1
  Divide_08384/1 -> Subtract_2d9ef/2
  State_psi_q_SG_D_6_163e7/1 -> Add_143fb/2
  Product_b1887/1 -> Subtract_75a6e/2
  Constant_R_a_3af7e/1 -> Product_6d514/1
  State_theta_SG_D_6_a7791/1 -> MathFunc_cos_41055/1
  MathFunc_cos_41055/1 -> Product_9e638/2
  Divide_fd7a5/1 -> Subtract_988de/1
  Product_9e638/1 -> Subtract_988de/2
  Input_v_q_SG_D_6_f6a8c/1 -> Product_b1887/1
  State_psi_d_SG_D_6_700ce/1 -> Product_37e9e/1
  Constant_pi_dab8a/1 -> Product_6be21/2
  Subtract_988de/1 -> Subtract_75a6e/1
  Product_6be21/1 -> Product_43aa7/1
  Product_43aa7/1 -> Product_23c04/1
  Divide_1b459/1 -> Add_fe05f/2
  Add_fe05f/1 -> Product_23c04/2
  Product_23c04/1 -> Blockout_d_psi_q_SG_D_6_609ad/1

== system IEEE14_case/SG_D_6/d_theta_SG_D_6_block ==
  note: d_theta_SG_D_6 in case14gfl
      | $w_{\mathrm{SG},D,6}-2\,\pi \,f_{0}$
      | Automatically generated on 2025-10-09 21:33:15 .
  State_w_SG_D_6_8d63a : Inport
  Add_57e97 : Sum
  Constant_-2.0_a62d6 : Constant  Value=-2.0
  Constant_f0_0b75f : Constant  Value=f0
  Constant_pi_5dca4 : Constant  Value=pi
  Product_42fbe : Product
  Product_6f3e9 : Product
  Blockout_d_theta_SG_D_6_40bf7 : Outport
  wires:
  Add_57e97/1 -> Blockout_d_theta_SG_D_6_40bf7/1
  Product_42fbe/1 -> Add_57e97/1
  Constant_-2.0_a62d6/1 -> Product_6f3e9/1
  Constant_pi_5dca4/1 -> Product_6f3e9/2
  Product_6f3e9/1 -> Product_42fbe/1
  Constant_f0_0b75f/1 -> Product_42fbe/2
  State_w_SG_D_6_8d63a/1 -> Add_57e97/2

== system IEEE14_case/SG_D_6/d_w_SG_D_6_block ==
  note: d_w_SG_D_6 in case14gfl
      | $\frac{2\,\pi \,T_{m,\mathrm{SG},D,6}\,f_{0}-D\,\left(w_{\mathrm{SG},D,6}-2\,\pi \,f_{0}\right)+2\,\pi \,f_{0}\,\left(\frac{\psi _{d,\mathrm{SG},D,6}\,\left(\psi _{q,\mathrm{SG},D,6}+\frac{\psi _{\mathrm{gq},\mathrm{SG},D,6}\,\left(x_{l}-x_{\mathrm{qdd}}\right)}{x_{l}-x_{\mathrm{qd}}}+\frac{\psi _{\mathrm{kq},\mathrm{SG},D,6}\,\left(x_{\mathrm{qd}}-x_{\mathrm{qdd}}\right)}{x_{l}-x_{\mathrm{qd}}}\right)}{x_{\mathrm{qdd}}}+\frac{\psi _{q,\mathrm{SG},D,6}\,\left(\frac{\psi _{\mathrm{1d},\mathrm{SG},D,6}\,\left(x_{\mathrm{dd}}-x_{\mathrm{ddd}}\right)}{x_{\mathrm{dd}}-x_{l}}-\psi _{d,\mathrm{SG},D,6}+\frac{\psi _{\mathrm{fd},\mathrm{SG},D,6}\,\left(x_{\mathrm{ddd}}-x_{l}\right)}{x_{\mathrm{dd}}-x_{l}}\right)}{x_{\mathrm{ddd}}}\right)}{2\,H}$
      | Automatically generated on 2025-10-09 21:33:14 .
  State_w_SG_D_6_3de25 : Inport
  State_T_m_SG_D_6_5b3c9 : Inport  Port=2
  State_psi_d_SG_D_6_61dab : Inport  Port=3
  State_psi_gq_SG_D_6_45419 : Inport  Port=4
  State_psi_kq_SG_D_6_9cfe6 : Inport  Port=5
  State_psi_q_SG_D_6_bcef0 : Inport  Port=6
  State_psi_q_SG_D_6_5e3e6 : Inport  Port=7
  State_psi_1d_SG_D_6_cbb96 : Inport  Port=8
  State_psi_d_SG_D_6_2f7e7 : Inport  Port=9
  State_psi_fd_SG_D_6_ba952 : Inport  Port=10
  Add_2dfe4 : Sum
  Add_3ab87 : Sum
  Add_3cb3a : Sum
  Add_61959 : Sum
  Add_ae3d8 : Sum
  Add_c9664 : Sum
  Add_e040d : Sum
  Add_e3c27 : Sum
  Constant_-1_5953e : Constant  Value=-1
  Constant_-1_8a66e : Constant  Value=-1
  Constant_-1_9ed88 : Constant  Value=-1
  Constant_-1_ba37d : Constant  Value=-1
  Constant_-1_e55d2 : Constant  Value=-1
  Constant_-1_e7fef : Constant  Value=-1
  Constant_-2.0_8e0e0 : Constant  Value=-2.0
  Constant_2.0_6d900 : Constant  Value=2.0
  Constant_2.0_9434a : Constant  Value=2.0
  Constant_2.0_dd79e : Constant  Value=2.0
  Constant_D_234f2 : Constant  Value=D
  Constant_H_fb415 : Constant  Value=H
  Constant_f0_41d6b : Constant  Value=f0
  Constant_f0_8d0a2 : Constant  Value=f0
  Constant_f0_fd0f8 : Constant  Value=f0
  Constant_pi_270e6 : Constant  Value=pi
  Constant_pi_4ba2e : Constant  Value=pi
  Constant_pi_a72ad : Constant  Value=pi
  Constant_x_dd_42e74 : Constant  Value=x_dd
  Constant_x_dd_cddac : Constant  Value=x_dd
  Constant_x_dd_ddf60 : Constant  Value=x_dd
  Constant_x_ddd_10f90 : Constant  Value=x_ddd
  Constant_x_ddd_b03bd : Constant  Value=x_ddd
  Constant_x_ddd_f1eee : Constant  Value=x_ddd
  Constant_x_l_057c9 : Constant  Value=x_l
  Constant_x_l_73c79 : Constant  Value=x_l
  Constant_x_l_81253 : Constant  Value=x_l
  Constant_x_l_8d252 : Constant  Value=x_l
  Constant_x_l_c924e : Constant  Value=x_l
  Constant_x_l_f02ea : Constant  Value=x_l
  Constant_x_qd_0cb8f : Constant  Value=x_qd
  Constant_x_qd_2c8a7 : Constant  Value=x_qd
  Constant_x_qd_333d9 : Constant  Value=x_qd
  Constant_x_qdd_3ffaa : Constant  Value=x_qdd
  Constant_x_qdd_5295f : Constant  Value=x_qdd
  Constant_x_qdd_fa4d1 : Constant  Value=x_qdd
  Divide_0d2b3 : Product  Inputs=*/
  Divide_3fbee : Product  Inputs=*/
  Divide_587d8 : Product  Inputs=*/
  Divide_73bca : Product  Inputs=*/
  Divide_d50dd : Product  Inputs=*/
  Divide_e565c : Product  Inputs=*/
  Divide_ee02f : Product  Inputs=*/
  Product_042db : Product
  Product_0c59d : Product
  Product_0e85d : Product
  Product_13f3d : Product
  Product_5b260 : Product
  Product_5c26c : Product
  Product_6589b : Product
  Product_6e8cd : Product
  Product_72353 : Product
  Product_769a5 : Product
  Product_7c30a : Product
  Product_809a0 : Product
  Product_8bf40 : Product
  Product_99360 : Product
  Product_9b525 : Product
  Product_9c5e6 : Product
  Product_bac4e : Product
  Product_e53d0 : Product
  Product_e9147 : Product
  Product_e942a : Product
  Product_f8858 : Product
  Product_fdcb7 : Product
  Subtract_13e9e : Sum  Inputs=+-
  Subtract_19e36 : Sum  Inputs=+-
  Subtract_37b50 : Sum  Inputs=+-
  Subtract_3cb50 : Sum  Inputs=+-
  Subtract_462cf : Sum  Inputs=+-
  Subtract_4f75b : Sum  Inputs=+-
  Subtract_727f7 : Sum  Inputs=+-
  Subtract_e2c26 : Sum  Inputs=+-
  Blockout_d_w_SG_D_6_858c2 : Outport
  wires:
  Constant_x_qd_2c8a7/1 -> Subtract_13e9e/1
  State_psi_d_SG_D_6_2f7e7/1 -> Add_61959/2
  Constant_x_l_8d252/1 -> Product_9b525/2
  Product_769a5/1 -> Product_7c30a/1
  Constant_-1_e55d2/1 -> Product_5c26c/1
  Constant_x_qdd_5295f/1 -> Add_3ab87/2
  Constant_f0_fd0f8/1 -> Product_0c59d/2
  Constant_x_qdd_fa4d1/1 -> Subtract_13e9e/2
  Constant_x_l_81253/1 -> Product_5c26c/2
  Product_5c26c/1 -> Add_3ab87/1
  Constant_-1_ba37d/1 -> Product_9b525/1
  Constant_x_qd_333d9/1 -> Add_ae3d8/2
  Constant_-1_9ed88/1 -> Product_809a0/1
  Constant_x_l_73c79/1 -> Product_809a0/2
  State_w_SG_D_6_3de25/1 -> Add_e040d/2
  Constant_-1_5953e/1 -> Product_72353/1
  Product_9b525/1 -> Add_2dfe4/1
  State_psi_1d_SG_D_6_cbb96/1 -> Product_72353/2
  Constant_x_dd_ddf60/1 -> Subtract_e2c26/1
  Subtract_37b50/1 -> Divide_0d2b3/2
  Add_2dfe4/1 -> Divide_73bca/2
  Constant_x_ddd_10f90/1 -> Subtract_e2c26/2
  State_psi_gq_SG_D_6_45419/1 -> Product_e53d0/1
  Constant_x_l_f02ea/1 -> Subtract_37b50/2
  Add_3ab87/1 -> Product_e53d0/2
  Constant_x_qd_0cb8f/1 -> Add_2dfe4/2
  State_psi_kq_SG_D_6_9cfe6/1 -> Product_0e85d/1
  Subtract_13e9e/1 -> Product_0e85d/2
  Constant_-1_8a66e/1 -> Product_769a5/1
  Product_809a0/1 -> Add_ae3d8/1
  Product_72353/1 -> Product_6589b/1
  Constant_-2.0_8e0e0/1 -> Product_13f3d/1
  Subtract_e2c26/1 -> Product_6589b/2
  Constant_x_dd_cddac/1 -> Subtract_37b50/1
  Constant_x_ddd_b03bd/1 -> Subtract_727f7/1
  Constant_x_l_057c9/1 -> Subtract_727f7/2
  Product_6589b/1 -> Divide_0d2b3/1
  Product_e53d0/1 -> Divide_73bca/1
  Product_0e85d/1 -> Divide_ee02f/1
  Add_ae3d8/1 -> Divide_ee02f/2
  Add_3cb3a/1 -> Subtract_3cb50/1
  Constant_2.0_6d900/1 -> Product_bac4e/1
  State_psi_fd_SG_D_6_ba952/1 -> Product_f8858/1
  Subtract_727f7/1 -> Product_f8858/2
  Constant_pi_270e6/1 -> Product_13f3d/2
  Constant_x_dd_42e74/1 -> Subtract_4f75b/1
  Constant_x_l_c924e/1 -> Subtract_4f75b/2
  Divide_0d2b3/1 -> Add_61959/1
  Divide_73bca/1 -> Subtract_462cf/1
  Product_f8858/1 -> Divide_3fbee/1
  Divide_ee02f/1 -> Subtract_462cf/2
  Subtract_4f75b/1 -> Divide_3fbee/2
  Product_0c59d/1 -> Add_e040d/1
  Constant_-1_e7fef/1 -> Product_6e8cd/1
  State_psi_d_SG_D_6_61dab/1 -> Product_6e8cd/2
  Add_61959/1 -> Subtract_19e36/1
  Subtract_462cf/1 -> Add_e3c27/1
  State_psi_q_SG_D_6_bcef0/1 -> Add_e3c27/2
  Divide_3fbee/1 -> Subtract_19e36/2
  Product_13f3d/1 -> Product_0c59d/1
  Constant_pi_4ba2e/1 -> Product_bac4e/2
  Product_6e8cd/1 -> Product_8bf40/1
  Subtract_19e36/1 -> Product_5b260/2
  Add_e3c27/1 -> Product_8bf40/2
  State_psi_q_SG_D_6_5e3e6/1 -> Product_5b260/1
  Constant_D_234f2/1 -> Product_769a5/2
  Product_bac4e/1 -> Product_e9147/1
  State_T_m_SG_D_6_5b3c9/1 -> Product_e9147/2
  Constant_2.0_dd79e/1 -> Product_99360/1
  Constant_pi_a72ad/1 -> Product_99360/2
  Product_8bf40/1 -> Divide_587d8/1
  Constant_x_qdd_3ffaa/1 -> Divide_587d8/2
  Product_5b260/1 -> Divide_e565c/1
  Constant_x_ddd_f1eee/1 -> Divide_e565c/2
  Add_e040d/1 -> Product_7c30a/2
  Product_e9147/1 -> Product_e942a/1
  Constant_f0_8d0a2/1 -> Product_e942a/2
  Product_99360/1 -> Product_042db/1
  Constant_f0_41d6b/1 -> Product_042db/2
  Divide_587d8/1 -> Add_c9664/1
  Divide_e565c/1 -> Add_c9664/2
  Product_7c30a/1 -> Add_3cb3a/1
  Product_e942a/1 -> Add_3cb3a/2
  Product_042db/1 -> Product_fdcb7/1
  Add_c9664/1 -> Product_fdcb7/2
  Product_fdcb7/1 -> Subtract_3cb50/2
  Constant_2.0_9434a/1 -> Product_9c5e6/1
  Constant_H_fb415/1 -> Product_9c5e6/2
  Subtract_3cb50/1 -> Divide_d50dd/1
  Product_9c5e6/1 -> Divide_d50dd/2
  Divide_d50dd/1 -> Blockout_d_w_SG_D_6_858c2/1

== system IEEE14_case/SG_D_6/i_d_SG_D_6_block ==
  note: i_d_SG_D_6 in case14gfl
      | $\frac{\sin\left(\theta _{\mathrm{SG},D,6}\right)\,\left(\frac{\psi _{\mathrm{1d},\mathrm{SG},D,6}\,\left(x_{\mathrm{dd}}-x_{\mathrm{ddd}}\right)}{x_{\mathrm{dd}}-x_{l}}-\psi _{d,\mathrm{SG},D,6}+\frac{\psi _{\mathrm{fd},\mathrm{SG},D,6}\,\left(x_{\mathrm{ddd}}-x_{l}\right)}{x_{\mathrm{dd}}-x_{l}}\right)}{x_{\mathrm{ddd}}}-\frac{\cos\left(\theta _{\mathrm{SG},D,6}\right)\,\left(\psi _{q,\mathrm{SG},D,6}+\frac{\psi _{\mathrm{gq},\mathrm{SG},D,6}\,\left(x_{l}-x_{\mathrm{qdd}}\right)}{x_{l}-x_{\mathrm{qd}}}+\frac{\psi _{\mathrm{kq},\mathrm{SG},D,6}\,\left(x_{\mathrm{qd}}-x_{\mathrm{qdd}}\right)}{x_{l}-x_{\mathrm{qd}}}\right)}{x_{\mathrm{qdd}}}$
      | Automatically generated on 2025-10-09 21:33:33 .
  State_psi_gq_SG_D_6_25250 : Inport
  State_psi_kq_SG_D_6_05164 : Inport  Port=2
  State_psi_q_SG_D_6_db020 : Inport  Port=3
  State_theta_SG_D_6_2ca6e : Inport  Port=4
  State_psi_1d_SG_D_6_32fc9 : Inport  Port=5
  State_psi_d_SG_D_6_8fce8 : Inport  Port=6
  State_psi_fd_SG_D_6_7efba : Inport  Port=7
  State_theta_SG_D_6_5c117 : Inport  Port=8
  Add_2130c : Sum
  Add_64d75 : Sum
  Add_6e550 : Sum
  Add_6f3d0 : Sum
  Add_ba97e : Sum
  Constant_-1_1ac78 : Constant  Value=-1
  Constant_-1_55283 : Constant  Value=-1
  Constant_-1_5652d : Constant  Value=-1
  Constant_-1_fa76f : Constant  Value=-1
  Constant_-1_fb37d : Constant  Value=-1
  Constant_x_dd_68927 : Constant  Value=x_dd
  Constant_x_dd_993b8 : Constant  Value=x_dd
  Constant_x_dd_c1731 : Constant  Value=x_dd
  Constant_x_ddd_480e1 : Constant  Value=x_ddd
  Constant_x_ddd_4c7c3 : Constant  Value=x_ddd
  Constant_x_ddd_d2b83 : Constant  Value=x_ddd
  Constant_x_l_41a62 : Constant  Value=x_l
  Constant_x_l_42383 : Constant  Value=x_l
  Constant_x_l_44865 : Constant  Value=x_l
  Constant_x_l_6a499 : Constant  Value=x_l
  Constant_x_l_94a58 : Constant  Value=x_l
  Constant_x_l_f63c1 : Constant  Value=x_l
  Constant_x_qd_0fec0 : Constant  Value=x_qd
  Constant_x_qd_9c34e : Constant  Value=x_qd
  Constant_x_qd_d0835 : Constant  Value=x_qd
  Constant_x_qdd_815f4 : Constant  Value=x_qdd
  Constant_x_qdd_a8440 : Constant  Value=x_qdd
  Constant_x_qdd_fd8f9 : Constant  Value=x_qdd
  Divide_552ff : Product  Inputs=*/
  Divide_73cdb : Product  Inputs=*/
  Divide_99815 : Product  Inputs=*/
  Divide_bd53d : Product  Inputs=*/
  Divide_f05fa : Product  Inputs=*/
  Divide_f993f : Product  Inputs=*/
  MathFunc_cos_5dbe0 : Trigonometry  Operator=cos
  MathFunc_sin_e2117 : Trigonometry
  Product_0727c : Product
  Product_25bd5 : Product
  Product_4b94f : Product
  Product_4fc42 : Product
  Product_54f9b : Product
  Product_68530 : Product
  Product_69cc3 : Product
  Product_7bbd1 : Product
  Product_98e21 : Product
  Product_c7153 : Product
  Product_f4b55 : Product
  Subtract_713e7 : Sum  Inputs=+-
  Subtract_88b70 : Sum  Inputs=+-
  Subtract_b7032 : Sum  Inputs=+-
  Subtract_e88a3 : Sum  Inputs=+-
  Subtract_e96b5 : Sum  Inputs=+-
  Subtract_e999b : Sum  Inputs=+-
  Subtract_eef8b : Sum  Inputs=+-
  Subtract_fb974 : Sum  Inputs=+-
  Blockout_i_d_SG_D_6_c0693 : Outport
  wires:
  Constant_x_qd_0fec0/1 -> Subtract_b7032/1
  Subtract_eef8b/1 -> Blockout_i_d_SG_D_6_c0693/1
  Subtract_fb974/1 -> Product_68530/2
  Constant_-1_5652d/1 -> Product_69cc3/1
  Subtract_e96b5/1 -> Product_7bbd1/1
  Constant_x_dd_c1731/1 -> Subtract_713e7/1
  Constant_x_qdd_fd8f9/1 -> Subtract_b7032/2
  Constant_x_l_6a499/1 -> Product_69cc3/2
  Divide_f05fa/1 -> Subtract_eef8b/1
  Add_6e550/1 -> Divide_bd53d/2
  Constant_x_l_94a58/1 -> Product_4fc42/2
  Constant_x_qdd_815f4/1 -> Add_64d75/2
  Product_69cc3/1 -> Add_64d75/1
  Constant_-1_1ac78/1 -> Product_4fc42/1
  Constant_-1_55283/1 -> Product_c7153/1
  Constant_x_l_41a62/1 -> Product_c7153/2
  State_psi_gq_SG_D_6_25250/1 -> Product_98e21/1
  Product_4b94f/1 -> Product_0727c/1
  Add_64d75/1 -> Product_98e21/2
  Constant_x_ddd_d2b83/1 -> Subtract_88b70/2
  Product_4fc42/1 -> Add_6e550/1
  Constant_x_qd_d0835/1 -> Add_6e550/2
  Constant_x_ddd_4c7c3/1 -> Divide_f993f/2
  State_psi_kq_SG_D_6_05164/1 -> Product_54f9b/1
  Product_f4b55/1 -> Divide_f05fa/1
  Subtract_b7032/1 -> Product_54f9b/2
  Product_c7153/1 -> Add_ba97e/1
  Constant_x_ddd_480e1/1 -> Subtract_fb974/1
  Constant_x_qd_9c34e/1 -> Add_ba97e/2
  Constant_-1_fb37d/1 -> Product_4b94f/1
  State_psi_fd_SG_D_6_7efba/1 -> Product_68530/1
  Product_54f9b/1 -> Divide_552ff/1
  State_psi_1d_SG_D_6_32fc9/1 -> Product_4b94f/2
  Product_68530/1 -> Divide_99815/1
  Constant_x_dd_68927/1 -> Subtract_88b70/1
  Product_98e21/1 -> Divide_bd53d/1
  Add_ba97e/1 -> Divide_552ff/2
  State_theta_SG_D_6_5c117/1 -> MathFunc_sin_e2117/1
  Subtract_88b70/1 -> Product_0727c/2
  Divide_73cdb/1 -> Add_6f3d0/1
  Constant_x_dd_993b8/1 -> Subtract_e88a3/1
  Constant_x_l_42383/1 -> Subtract_e88a3/2
  Subtract_e999b/1 -> Add_2130c/1
  Constant_x_l_f63c1/1 -> Subtract_fb974/2
  Divide_bd53d/1 -> Subtract_e999b/1
  Divide_552ff/1 -> Subtract_e999b/2
  Product_0727c/1 -> Divide_73cdb/1
  Subtract_e88a3/1 -> Divide_73cdb/2
  Constant_-1_fa76f/1 -> Product_25bd5/1
  Constant_x_l_44865/1 -> Subtract_713e7/2
  MathFunc_cos_5dbe0/1 -> Product_f4b55/2
  State_psi_q_SG_D_6_db020/1 -> Add_2130c/2
  State_psi_d_SG_D_6_8fce8/1 -> Add_6f3d0/2
  Subtract_713e7/1 -> Divide_99815/2
  Add_2130c/1 -> Product_25bd5/2
  State_theta_SG_D_6_2ca6e/1 -> MathFunc_cos_5dbe0/1
  Add_6f3d0/1 -> Subtract_e96b5/1
  Divide_99815/1 -> Subtract_e96b5/2
  Product_25bd5/1 -> Product_f4b55/1
  MathFunc_sin_e2117/1 -> Product_7bbd1/2
  Constant_x_qdd_a8440/1 -> Divide_f05fa/2
  Product_7bbd1/1 -> Divide_f993f/1
  Divide_f993f/1 -> Subtract_eef8b/2
